simulink model "simullink_controller"  (R2016a)
settings: Solver=VariableStepAuto  StartTime=0.0  StopTime=20  MaxStep=0.01  RelTol=1e-4
settings Model: Creator=kreitzem  LastModifiedBy=kreitzem
settings DataIOCC: LimitDataPoints=on  SaveOutput=off  SaveTime=off
settings OptimizationCC: ExpressionDepthLimit=2147483647  LifeSpan=1
settings DebuggingCC: UnderspecifiedInitializationDetection=Classic  MergeDetectMultiDrivingBlocksExec=none  FcnCallInpInsideContextMsg=EnableAllAsWarning  AllowSymbolicDim=off  StateNameClashWarn=warning
settings GRTTargetCC: CombineOutputUpdateFcns=off  GRTInterface=on

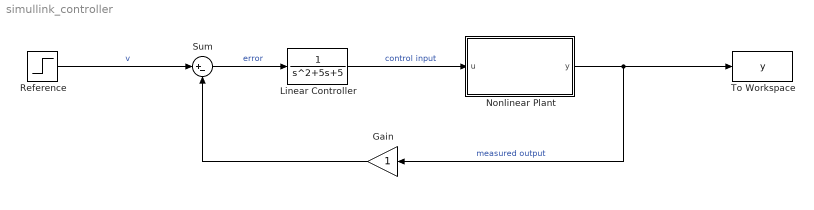
== system simullink_controller ==
  Gain : Gain
  Linear Controller : TransferFcn  Denominator=[1 5 5]
  Nonlinear Plant : Subsystem
  Reference : Step  SampleTime=0
  Sum : Sum  Inputs=|+-
  To Workspace : ToWorkspace  VariableName=y  SaveFormat=Timeseries  SampleTime=-1
  wires:
  Reference/1 -> Sum/1  "v"
  Nonlinear Plant/1(y) -> To Workspace/1, Gain/1  "measured output"
  Sum/1 -> Linear Controller/1  "error"
  Linear Controller/1 -> Nonlinear Plant/1(u)  "control input"
  Gain/1 -> Sum/2

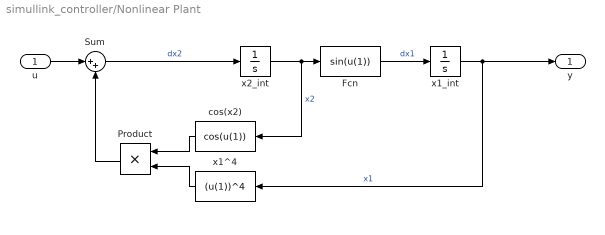
== system simullink_controller/Nonlinear Plant ==
  u : Inport
  Fcn : Fcn  Expr=sin(u(1))
  Product : Product
  Sum : Sum  Inputs=|++
  cos(x2) : Fcn  Expr=cos(u(1))
  x1^4 : Fcn  Expr=(u(1))^4
  x1_int : Integrator
  x2_int : Integrator
  y : Outport
  wires:
  x1_int/1 -> x1^4/1, y/1  "x1"
  Fcn/1 -> x1_int/1  "dx1"
  x2_int/1 -> cos(x2)/1, Fcn/1  "x2"
  u/1 -> Sum/1
  Product/1 -> Sum/2
  Sum/1 -> x2_int/1  "dx2"
  cos(x2)/1 -> Product/1
  x1^4/1 -> Product/2
